simulink library "Iphone15_battery"  (R2025a)
settings: Solver=VariableStepAuto  StartTime=0.0  StopTime=10.0  RelTol=1e-3
undefined symbols (not defined in the file or in its folder): battery_builder_rtmsupport, gcbh
libraries: Iphone15_battery_lib x2
settings Model: Creator=andre  LastModifiedBy=andre

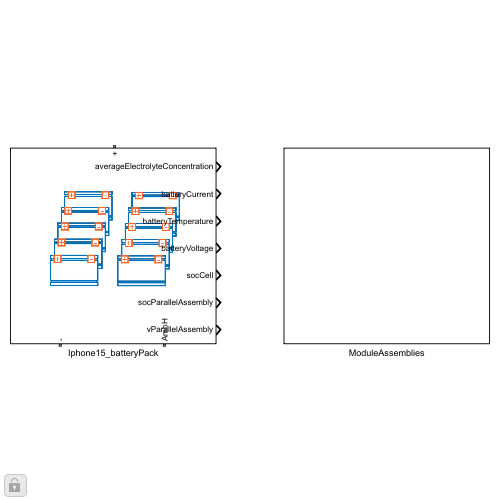
[thumbnail: Simulink's stored preview of the top-level diagram]
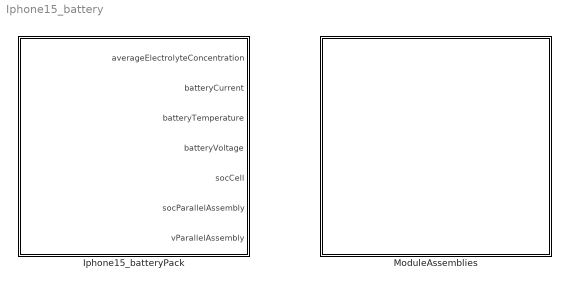
== system Iphone15_battery ==
  Iphone15_batteryPack : Subsystem  LoadFcn=battery_builder_rtmsupport('loadfcn',gcbh);
      settings: CopyFcn=battery_builder_rtmsupport('copyfcn',gcbh);  PreCopyFcn=battery_builder_rtmsupport('precopyfcn',gcbh);  PreDeleteFcn=battery_builder_rtmsupport('predeletefcn',gcbh);  PortSchema="{\"entries\":[{\"content\":{\"sides\":[{\"content\":{\"connectorIds\":[\"LConn1\"]},\"type\":\"ConnectorPlacement.EquallySpacedRectSide\",\"uuid\":\"2608078c-e1aa-41b5-833c-c2e701ab0cab\"},{\"content\":{\"connectorIds\":[\"RConn1\",\"RConn2\"],\"side\":\"RIGHT\"},\"type\":\"ConnectorPlacement.EquallySpacedRectSide\",\"uuid\":\"d1338bb5-d28d-4189-96be-004d18f9ecfd\"},{\"content\":{\"side\":\"TOP\"},\"type\":\"ConnectorPlacement.EquallySpacedRectSide\",\"uuid\":\"07cf85c3-a5da-4c34-90eb-ff605cc69d48\"},{\"content\":{\"connectorIds\":[\"Out1\",\"Out2\",\"Out3\",\"Out4\",\"Out5\",\"Out6\",\"Out7\"],\"side\":\"BOTTOM\"},\"type\":\"ConnectorPlacement.EquallySpacedRectSide\",\"uuid\":\"789138ec-b892-4716-bd54-c98053e62821\"}]},\"type\":\"ConnectorPlacement.EquallySpacedConnector\",\"uuid\":\"c3353730-e649-4a82-9e2e-d21f518e46da\"}],\"packageUris\":[\"http://schema.mathworks.com/mf0/Connector/R2020b\"],\"version\":\"1.0\"}"
      mask Display: image('$imagefile')
  ModuleAssemblies : Subsystem

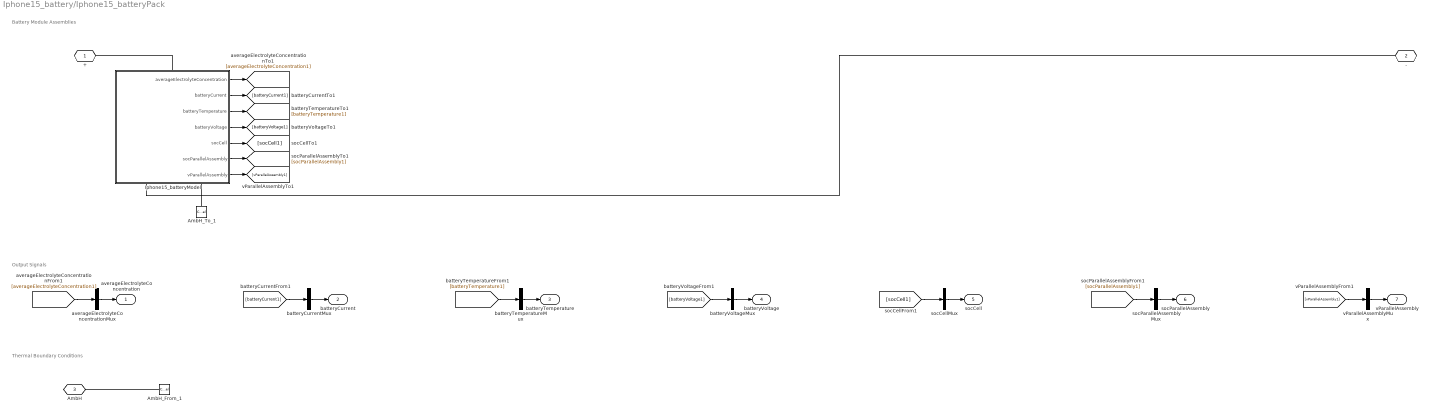
== system Iphone15_battery/Iphone15_batteryPack ==
  note: Battery Module Assemblies
  note: Output Signals
  note: Thermal Boundary Conditions
  AmbH_From_1 : ConnectionLabel  Label=ambH_1
  AmbH_To_1 : ConnectionLabel  Label=ambH_1
  Iphone15_batteryModel : Subsystem  LoadFcn=battery_builder_rtmsupport('loadfcn',gcbh);
      settings: CopyFcn=battery_builder_rtmsupport('copyfcn',gcbh);  PreCopyFcn=battery_builder_rtmsupport('precopyfcn',gcbh);  PreDeleteFcn=battery_builder_rtmsupport('predeletefcn',gcbh);  PortSchema="{\"entries\":[{\"content\":{\"sides\":[{\"content\":{\"connectorIds\":[\"LConn1\"]},\"type\":\"ConnectorPlacement.EquallySpacedRectSide\",\"uuid\":\"2608078c-e1aa-41b5-833c-c2e701ab0cab\"},{\"content\":{\"connectorIds\":[\"RConn1\",\"RConn2\"],\"side\":\"RIGHT\"},\"type\":\"ConnectorPlacement.EquallySpacedRectSide\",\"uuid\":\"d1338bb5-d28d-4189-96be-004d18f9ecfd\"},{\"content\":{\"side\":\"TOP\"},\"type\":\"ConnectorPlacement.EquallySpacedRectSide\",\"uuid\":\"07cf85c3-a5da-4c34-90eb-ff605cc69d48\"},{\"content\":{\"connectorIds\":[\"Out1\",\"Out2\",\"Out3\",\"Out4\",\"Out5\",\"Out6\",\"Out7\"],\"side\":\"BOTTOM\"},\"type\":\"ConnectorPlacement.EquallySpacedRectSide\",\"uuid\":\"e3e1380c-838f-41f2-8f13-742e9e0e9750\"}]},\"type\":\"ConnectorPlacement.EquallySpacedConnector\",\"uuid\":\"c3353730-e649-4a82-9e2e-d21f518e46da\"}],\"packageUris\":[\"http://schema.mathworks.com/mf0/Connector/R2020b\"],\"version\":\"1.0\"}"
      mask Display: image('$imagefile')
  averageElectrolyteConcentrationMux : Mux  Inputs=1
  batteryCurrentMux : Mux  Inputs=1
  batteryTemperatureMux : Mux  Inputs=1
  batteryVoltageMux : Mux  Inputs=1
  socCellMux : Mux  Inputs=1
  socParallelAssemblyMux : Mux  Inputs=1
  vParallelAssemblyMux : Mux  Inputs=1
  + : PMIOPort  Side=Left
  - : PMIOPort  Port=2  Side=Right
  AmbH : PMIOPort  Port=3  Side=Right  ConnectionType=Connection: foundation.thermal.thermal
  averageElectrolyteConcentration : Outport
  batteryCurrent : Outport  Port=2
  batteryTemperature : Outport  Port=3
  batteryVoltage : Outport  Port=4
  socCell : Outport  Port=5
  socParallelAssembly : Outport  Port=6
  vParallelAssembly : Outport  Port=7
  wires:
  Iphone15_batteryModel/1(averageElectrolyteConcentration) -> [averageElectrolyteConcentration1]
  averageElectrolyteConcentrationMux/1 -> averageElectrolyteConcentration/1
  [averageElectrolyteConcentration1] -> averageElectrolyteConcentrationMux/1
  Iphone15_batteryModel/2(batteryCurrent) -> [batteryCurrent1]
  batteryCurrentMux/1 -> batteryCurrent/1
  [batteryCurrent1] -> batteryCurrentMux/1
  Iphone15_batteryModel/3(batteryTemperature) -> [batteryTemperature1]
  batteryTemperatureMux/1 -> batteryTemperature/1
  [batteryTemperature1] -> batteryTemperatureMux/1
  Iphone15_batteryModel/4(batteryVoltage) -> [batteryVoltage1]
  batteryVoltageMux/1 -> batteryVoltage/1
  [batteryVoltage1] -> batteryVoltageMux/1
  Iphone15_batteryModel/5(socCell) -> [socCell1]
  socCellMux/1 -> socCell/1
  [socCell1] -> socCellMux/1
  Iphone15_batteryModel/6(socParallelAssembly) -> [socParallelAssembly1]
  socParallelAssemblyMux/1 -> socParallelAssembly/1
  [socParallelAssembly1] -> socParallelAssemblyMux/1
  Iphone15_batteryModel/7(vParallelAssembly) -> [vParallelAssembly1]
  vParallelAssemblyMux/1 -> vParallelAssembly/1
  [vParallelAssembly1] -> vParallelAssemblyMux/1
  connections:
  Iphone15_batteryModel/LConn1 -- +/RConn1
  Iphone15_batteryModel/RConn1 -- -/RConn1
  AmbH_To_1/LConn1 -- Iphone15_batteryModel/RConn2
  AmbH_From_1/LConn1 -- AmbH/RConn1

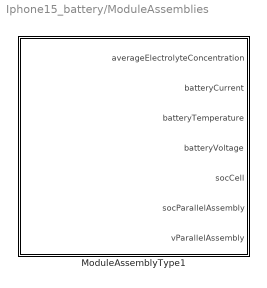
== system Iphone15_battery/ModuleAssemblies ==
  ModuleAssemblyType1 : Subsystem  LoadFcn=battery_builder_rtmsupport('loadfcn',gcbh);
      settings: CopyFcn=battery_builder_rtmsupport('copyfcn',gcbh);  PreCopyFcn=battery_builder_rtmsupport('precopyfcn',gcbh);  PreDeleteFcn=battery_builder_rtmsupport('predeletefcn',gcbh);  PortSchema="{\"entries\":[{\"content\":{\"sides\":[{\"content\":{\"connectorIds\":[\"LConn1\"]},\"type\":\"ConnectorPlacement.EquallySpacedRectSide\",\"uuid\":\"2608078c-e1aa-41b5-833c-c2e701ab0cab\"},{\"content\":{\"connectorIds\":[\"RConn1\",\"RConn2\"],\"side\":\"RIGHT\"},\"type\":\"ConnectorPlacement.EquallySpacedRectSide\",\"uuid\":\"d1338bb5-d28d-4189-96be-004d18f9ecfd\"},{\"content\":{\"side\":\"TOP\"},\"type\":\"ConnectorPlacement.EquallySpacedRectSide\",\"uuid\":\"07cf85c3-a5da-4c34-90eb-ff605cc69d48\"},{\"content\":{\"connectorIds\":[\"Out1\",\"Out2\",\"Out3\",\"Out4\",\"Out5\",\"Out6\",\"Out7\"],\"side\":\"BOTTOM\"},\"type\":\"ConnectorPlacement.EquallySpacedRectSide\",\"uuid\":\"e3e1380c-838f-41f2-8f13-742e9e0e9750\"}]},\"type\":\"ConnectorPlacement.EquallySpacedConnector\",\"uuid\":\"c3353730-e649-4a82-9e2e-d21f518e46da\"}],\"packageUris\":[\"http://schema.mathworks.com/mf0/Connector/R2020b\"],\"version\":\"1.0\"}"
      mask Display: image('$imagefile')

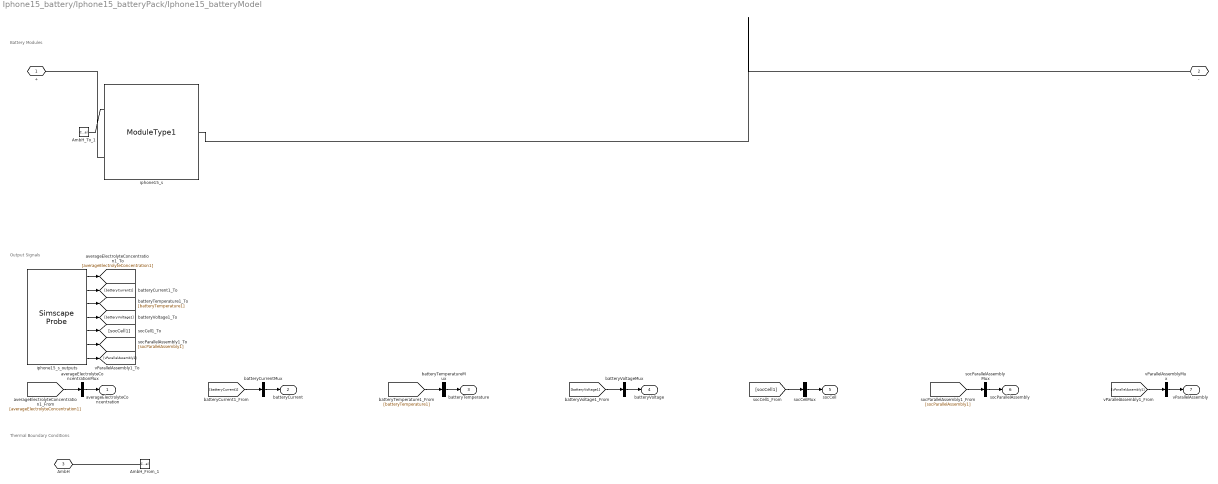
== system Iphone15_battery/Iphone15_batteryPack/Iphone15_batteryModel ==
  note: Thermal Boundary Conditions
  note: Output Signals
  note: Battery Modules
  AmbH_From_1 : ConnectionLabel  Label=ambH_1
  AmbH_To_1 : ConnectionLabel  Label=ambH_1
  averageElectrolyteConcentrationMux : Mux  Inputs=1
  batteryCurrentMux : Mux  Inputs=1
  batteryTemperatureMux : Mux  Inputs=1
  batteryVoltageMux : Mux  Inputs=1
  iphone15_s : Iphone15_battery_lib/Modules/ModuleType1  ExtrapolationMethodCell=simscape.enum.extrapolation.nearest  ThicknessAnodeCell=3.4E-5 m  ElectrolyteLayerCountAnodeCell=10  ThicknessSeparatorCell=2.5E-5 m  ElectrolyteLayerCountSeparatorCell=5  ThicknessCathodeCell=8E-5 m  ElectrolyteLayerCountCathodeCell=10  ElectrodePlateAreaCell=1.8E-1 m^2  ParticleRadiusAnodeCell=5E-6 m  ShellCountAnodeCell=10  ParticleRadiusCathodeCell=5E-8 m  ShellCountCathodeCell=10  ActiveMaterialVolumeFractionAnodeCell=0.58  ActiveMaterialVolumeFractionCathodeCell=0.374  NormalizedStoichiometryBreakpointsCell=linspace(0.025, 0.975, 39)  OpenCircuitPotentialAnodeCell=[.435; .325; .259; .221; .204; .194; .179; .166; .155; .145; .137; .131; .128; .127; .126; .125; .124; .123; .122; .121; .118; .117; .112; .109; .105; .1; .098; .095; .094; .093; .091; .09; .089; .088; .087; .086; .085; .084; .083] V  OpenCircuitPotentialCathodeCell=[3.598; 3.53; 3.494; 3.474; 3.46; 3.455; 3.454; 3.453; 3.4528; 3.4526; 3.4524; 3.452; 3.4518; 3.4516; 3.4514; 3.4512; 3.451; 3.4508; 3.4506; 3.4503; 3.45; 3.4498; 3.4495; 3.4493; 3.449; 3.4488; 3.4486; 3.4484; 3.4482; 3.4479; 3.4477; 3.4475; 3.4473; 3.447; 3.4468; 3.4466; 3.4464; 3.4462; 3.4458] V  MaximumConcentrationAnodeCell=30555 mol/m^3  MaximumStoichiometryAnodeCell=0.811  MinimumStoichiometryAnodeCell=0.0132  MaximumConcentrationCathodeCell=22806 mol/m^3  MaximumStoichiometryCathodeCell=0.74  MinimumStoichiometryCathodeCell=0.035  ActiveMaterialDiffusionCoefficientAnodeCell=3E-15 m^2/s  ActiveMaterialDiffusionCoefficientCathodeCell=5.9E-20 m^2/s  ConductivityAnodeCell=100 S/m  ConductivityCathodeCell=0.5 S/m  CurrentCollectorResistanceCell=0 Ohm  ElectrolyteVolumeFractionAnodeCell=0.3874  ElectrolyteVolumeFractionSeparatorCell=0.45  ElectrolyteVolumeFractionCathodeCell=0.5725  ElectrolyteConductivityCell=0.29 S/m  BruggemanExponentAnodeCell=1.5  BruggemanExponentSeparatorCell=1.5  BruggemanExponentCathodeCell=1.5  TransferenceNumberCell=0.363  ElectrolyteDiffusionCoefficientCell=2E-10 m^2/s  ChargeTransferRateAnodeCell=8.8E-11 m^(5/2)/(mol^(1/2)*s)  ChargeTransferRateCathodeCell=2.8E-13 m^(5/2)/(mol^(1/2)*s)  BatteryThermalMassCell=77 J/K  ArrheniusReferenceTemperatureCell=298.15 K  ActiveMaterialDiffusionActivationEnergyAnodeCell=39000 J/mol  ActiveMaterialDiffusionActivationEnergyCathodeCell=35000 J/mol  ElectrolyteDiffusionActivationEnergyCell=26600 J/mol  ConductivityActivationEnergyAnodeCell=3000 J/mol  ConductivityActivationEnergyCathodeCell=3000 J/mol  ElectrolyteConductivityActivationEnergyCell=11000 J/mol  ChargeTransferActivationEnergyAnodeCell=13000 J/mol  ChargeTransferActivationEnergyCathodeCell=20000 J/mol  AmbientResistance=25 K/W  P=1  S=1  batteryCurrent_specify=off  batteryCurrent_priority=None  batteryCurrent=0 A  batteryCurrent_nominal_specify=off  batteryCurrent_nominal_value=1  batteryCurrent_nominal_unit=A  batteryVoltage_specify=off  batteryVoltage_priority=None  batteryVoltage=0 V  batteryVoltage_nominal_specify=off  batteryVoltage_nominal_value=1  batteryVoltage_nominal_unit=V  averageElectrolyteConcentration_specify=off  averageElectrolyteConcentration_priority=High  averageElectrolyteConcentration=1200 mol/m^3  averageElectrolyteConcentration_nominal_specify=off  averageElectrolyteConcentration_nominal_value=1  averageElectrolyteConcentration_nominal_unit=mol/m^3  socCell_specify=off  socCell_priority=High  socCell=0.5  socCell_nominal_specify=off  socCell_nominal_value=1  socCell_nominal_unit=1  batteryTemperature_specify=off  batteryTemperature_priority=High  batteryTemperature=298.15 K  batteryTemperature_nominal_specify=off  batteryTemperature_nominal_value=1  batteryTemperature_nominal_unit=K  vParallelAssembly_specify=off  vParallelAssembly_priority=None  vParallelAssembly=0 V  vParallelAssembly_nominal_specify=off  vParallelAssembly_nominal_value=1  vParallelAssembly_nominal_unit=V  socParallelAssembly_specify=off  socParallelAssembly_priority=None  socParallelAssembly=1  socParallelAssembly_nominal_specify=off  socParallelAssembly_nominal_value=1  socParallelAssembly_nominal_unit=1
      settings: InternalSimscapePortConfiguration="{\"Bottom\":[{\"id\":\"n\",\"label\":\"-\",\"type\":\"foundation.electrical.electrical\"}],\"Left\":[{\"id\":\"AmbH\",\"label\":\"AmbH\",\"type\":\"foundation.thermal.thermal\"}],\"Right\":[],\"Top\":[{\"id\":\"p\",\"label\":\"+\",\"type\":\"foundation.electrical.electrical\"}]}"
  iphone15_s_outputs : SimscapeProbe  BoundBlock=57  Variables="{\"averageElectrolyteConcentration\":{\"Probing\":\"ON\"},\"batteryCurrent\":{\"Probing\":\"ON\"},\"batteryTemperature\":{\"Probing\":\"ON\"},\"batteryVoltage\":{\"Probing\":\"ON\"},\"socCell\":{\"Probing\":\"ON\"},\"socParallelAssembly\":{\"Probing\":\"ON\"},\"vParallelAssembly\":{\"Probing\":\"ON\"}}"
  socCellMux : Mux  Inputs=1
  socParallelAssemblyMux : Mux  Inputs=1
  vParallelAssemblyMux : Mux  Inputs=1
  + : PMIOPort  Side=Left
  - : PMIOPort  Port=2  Side=Right
  AmbH : PMIOPort  Port=3  Side=Right  ConnectionType=Connection: foundation.thermal.thermal
  averageElectrolyteConcentration : Outport
  batteryCurrent : Outport  Port=2
  batteryTemperature : Outport  Port=3
  batteryVoltage : Outport  Port=4
  socCell : Outport  Port=5
  socParallelAssembly : Outport  Port=6
  vParallelAssembly : Outport  Port=7
  wires:
  [vParallelAssembly1] -> vParallelAssemblyMux/1
  vParallelAssemblyMux/1 -> vParallelAssembly/1
  iphone15_s_outputs/7 -> [vParallelAssembly1]
  [socParallelAssembly1] -> socParallelAssemblyMux/1
  socParallelAssemblyMux/1 -> socParallelAssembly/1
  iphone15_s_outputs/6 -> [socParallelAssembly1]
  [socCell1] -> socCellMux/1
  socCellMux/1 -> socCell/1
  iphone15_s_outputs/5 -> [socCell1]
  [batteryVoltage1] -> batteryVoltageMux/1
  batteryVoltageMux/1 -> batteryVoltage/1
  iphone15_s_outputs/4 -> [batteryVoltage1]
  [batteryTemperature1] -> batteryTemperatureMux/1
  batteryTemperatureMux/1 -> batteryTemperature/1
  iphone15_s_outputs/3 -> [batteryTemperature1]
  [batteryCurrent1] -> batteryCurrentMux/1
  batteryCurrentMux/1 -> batteryCurrent/1
  iphone15_s_outputs/2 -> [batteryCurrent1]
  [averageElectrolyteConcentration1] -> averageElectrolyteConcentrationMux/1
  averageElectrolyteConcentrationMux/1 -> averageElectrolyteConcentration/1
  iphone15_s_outputs/1 -> [averageElectrolyteConcentration1]
  connections:
  AmbH_From_1/LConn1 -- AmbH/RConn1
  AmbH_To_1/LConn1 -- iphone15_s/LConn1
  iphone15_s/RConn1 -- -/RConn1
  iphone15_s/LConn2 -- +/RConn1

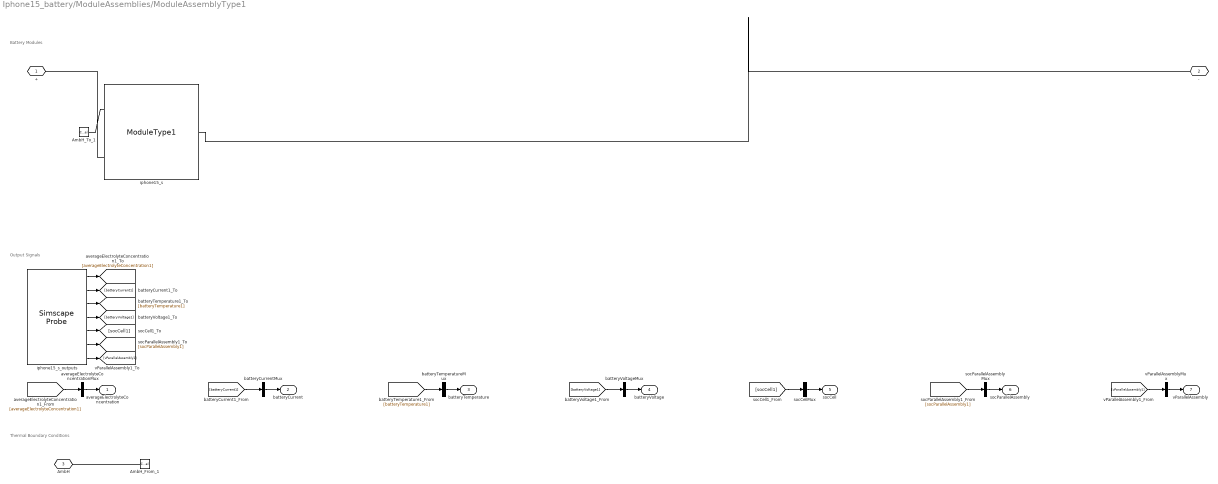
== system Iphone15_battery/ModuleAssemblies/ModuleAssemblyType1 ==
  note: Battery Modules
  note: Output Signals
  note: Thermal Boundary Conditions
  AmbH_From_1 : ConnectionLabel  Label=ambH_1
  AmbH_To_1 : ConnectionLabel  Label=ambH_1
  averageElectrolyteConcentrationMux : Mux  Inputs=1
  batteryCurrentMux : Mux  Inputs=1
  batteryTemperatureMux : Mux  Inputs=1
  batteryVoltageMux : Mux  Inputs=1
  iphone15_s : Iphone15_battery_lib/Modules/ModuleType1  ExtrapolationMethodCell=simscape.enum.extrapolation.nearest  ThicknessAnodeCell=3.4E-5 m  ElectrolyteLayerCountAnodeCell=10  ThicknessSeparatorCell=2.5E-5 m  ElectrolyteLayerCountSeparatorCell=5  ThicknessCathodeCell=8E-5 m  ElectrolyteLayerCountCathodeCell=10  ElectrodePlateAreaCell=1.8E-1 m^2  ParticleRadiusAnodeCell=5E-6 m  ShellCountAnodeCell=10  ParticleRadiusCathodeCell=5E-8 m  ShellCountCathodeCell=10  ActiveMaterialVolumeFractionAnodeCell=0.58  ActiveMaterialVolumeFractionCathodeCell=0.374  NormalizedStoichiometryBreakpointsCell=linspace(0.025, 0.975, 39)  OpenCircuitPotentialAnodeCell=[.435; .325; .259; .221; .204; .194; .179; .166; .155; .145; .137; .131; .128; .127; .126; .125; .124; .123; .122; .121; .118; .117; .112; .109; .105; .1; .098; .095; .094; .093; .091; .09; .089; .088; .087; .086; .085; .084; .083] V  OpenCircuitPotentialCathodeCell=[3.598; 3.53; 3.494; 3.474; 3.46; 3.455; 3.454; 3.453; 3.4528; 3.4526; 3.4524; 3.452; 3.4518; 3.4516; 3.4514; 3.4512; 3.451; 3.4508; 3.4506; 3.4503; 3.45; 3.4498; 3.4495; 3.4493; 3.449; 3.4488; 3.4486; 3.4484; 3.4482; 3.4479; 3.4477; 3.4475; 3.4473; 3.447; 3.4468; 3.4466; 3.4464; 3.4462; 3.4458] V  MaximumConcentrationAnodeCell=30555 mol/m^3  MaximumStoichiometryAnodeCell=0.811  MinimumStoichiometryAnodeCell=0.0132  MaximumConcentrationCathodeCell=22806 mol/m^3  MaximumStoichiometryCathodeCell=0.74  MinimumStoichiometryCathodeCell=0.035  ActiveMaterialDiffusionCoefficientAnodeCell=3E-15 m^2/s  ActiveMaterialDiffusionCoefficientCathodeCell=5.9E-20 m^2/s  ConductivityAnodeCell=100 S/m  ConductivityCathodeCell=0.5 S/m  CurrentCollectorResistanceCell=0 Ohm  ElectrolyteVolumeFractionAnodeCell=0.3874  ElectrolyteVolumeFractionSeparatorCell=0.45  ElectrolyteVolumeFractionCathodeCell=0.5725  ElectrolyteConductivityCell=0.29 S/m  BruggemanExponentAnodeCell=1.5  BruggemanExponentSeparatorCell=1.5  BruggemanExponentCathodeCell=1.5  TransferenceNumberCell=0.363  ElectrolyteDiffusionCoefficientCell=2E-10 m^2/s  ChargeTransferRateAnodeCell=8.8E-11 m^(5/2)/(mol^(1/2)*s)  ChargeTransferRateCathodeCell=2.8E-13 m^(5/2)/(mol^(1/2)*s)  BatteryThermalMassCell=77 J/K  ArrheniusReferenceTemperatureCell=298.15 K  ActiveMaterialDiffusionActivationEnergyAnodeCell=39000 J/mol  ActiveMaterialDiffusionActivationEnergyCathodeCell=35000 J/mol  ElectrolyteDiffusionActivationEnergyCell=26600 J/mol  ConductivityActivationEnergyAnodeCell=3000 J/mol  ConductivityActivationEnergyCathodeCell=3000 J/mol  ElectrolyteConductivityActivationEnergyCell=11000 J/mol  ChargeTransferActivationEnergyAnodeCell=13000 J/mol  ChargeTransferActivationEnergyCathodeCell=20000 J/mol  AmbientResistance=25 K/W  P=1  S=1  batteryCurrent_specify=off  batteryCurrent_priority=None  batteryCurrent=0 A  batteryCurrent_nominal_specify=off  batteryCurrent_nominal_value=1  batteryCurrent_nominal_unit=A  batteryVoltage_specify=off  batteryVoltage_priority=None  batteryVoltage=0 V  batteryVoltage_nominal_specify=off  batteryVoltage_nominal_value=1  batteryVoltage_nominal_unit=V  averageElectrolyteConcentration_specify=off  averageElectrolyteConcentration_priority=High  averageElectrolyteConcentration=1200 mol/m^3  averageElectrolyteConcentration_nominal_specify=off  averageElectrolyteConcentration_nominal_value=1  averageElectrolyteConcentration_nominal_unit=mol/m^3  socCell_specify=off  socCell_priority=High  socCell=0.5  socCell_nominal_specify=off  socCell_nominal_value=1  socCell_nominal_unit=1  batteryTemperature_specify=off  batteryTemperature_priority=High  batteryTemperature=298.15 K  batteryTemperature_nominal_specify=off  batteryTemperature_nominal_value=1  batteryTemperature_nominal_unit=K  vParallelAssembly_specify=off  vParallelAssembly_priority=None  vParallelAssembly=0 V  vParallelAssembly_nominal_specify=off  vParallelAssembly_nominal_value=1  vParallelAssembly_nominal_unit=V  socParallelAssembly_specify=off  socParallelAssembly_priority=None  socParallelAssembly=1  socParallelAssembly_nominal_specify=off  socParallelAssembly_nominal_value=1  socParallelAssembly_nominal_unit=1
      settings: InternalSimscapePortConfiguration="{\"Bottom\":[{\"id\":\"n\",\"label\":\"-\",\"type\":\"foundation.electrical.electrical\"}],\"Left\":[{\"id\":\"AmbH\",\"label\":\"AmbH\",\"type\":\"foundation.thermal.thermal\"}],\"Right\":[],\"Top\":[{\"id\":\"p\",\"label\":\"+\",\"type\":\"foundation.electrical.electrical\"}]}"
  iphone15_s_outputs : SimscapeProbe  BoundBlock=3  Variables="{\"averageElectrolyteConcentration\":{\"Probing\":\"ON\"},\"batteryCurrent\":{\"Probing\":\"ON\"},\"batteryTemperature\":{\"Probing\":\"ON\"},\"batteryVoltage\":{\"Probing\":\"ON\"},\"socCell\":{\"Probing\":\"ON\"},\"socParallelAssembly\":{\"Probing\":\"ON\"},\"vParallelAssembly\":{\"Probing\":\"ON\"}}"
  socCellMux : Mux  Inputs=1
  socParallelAssemblyMux : Mux  Inputs=1
  vParallelAssemblyMux : Mux  Inputs=1
  + : PMIOPort  Side=Left
  - : PMIOPort  Port=2  Side=Right
  AmbH : PMIOPort  Port=3  Side=Right  ConnectionType=Connection: foundation.thermal.thermal
  averageElectrolyteConcentration : Outport
  batteryCurrent : Outport  Port=2
  batteryTemperature : Outport  Port=3
  batteryVoltage : Outport  Port=4
  socCell : Outport  Port=5
  socParallelAssembly : Outport  Port=6
  vParallelAssembly : Outport  Port=7
  wires:
  iphone15_s_outputs/1 -> [averageElectrolyteConcentration1]
  averageElectrolyteConcentrationMux/1 -> averageElectrolyteConcentration/1
  [averageElectrolyteConcentration1] -> averageElectrolyteConcentrationMux/1
  iphone15_s_outputs/2 -> [batteryCurrent1]
  batteryCurrentMux/1 -> batteryCurrent/1
  [batteryCurrent1] -> batteryCurrentMux/1
  iphone15_s_outputs/3 -> [batteryTemperature1]
  batteryTemperatureMux/1 -> batteryTemperature/1
  [batteryTemperature1] -> batteryTemperatureMux/1
  iphone15_s_outputs/4 -> [batteryVoltage1]
  batteryVoltageMux/1 -> batteryVoltage/1
  [batteryVoltage1] -> batteryVoltageMux/1
  iphone15_s_outputs/5 -> [socCell1]
  socCellMux/1 -> socCell/1
  [socCell1] -> socCellMux/1
  iphone15_s_outputs/6 -> [socParallelAssembly1]
  socParallelAssemblyMux/1 -> socParallelAssembly/1
  [socParallelAssembly1] -> socParallelAssemblyMux/1
  iphone15_s_outputs/7 -> [vParallelAssembly1]
  vParallelAssemblyMux/1 -> vParallelAssembly/1
  [vParallelAssembly1] -> vParallelAssemblyMux/1
  connections:
  iphone15_s/LConn2 -- +/RConn1
  iphone15_s/RConn1 -- -/RConn1
  AmbH_To_1/LConn1 -- iphone15_s/LConn1
  AmbH_From_1/LConn1 -- AmbH/RConn1
